simulink library "tether002_ul"  (R2020a)
settings: Solver=VariableStepAuto  StartTime=0.0  StopTime=10.0  RelTol=1e-3
values from neighbouring files (symbols this model uses):
  initNodePos = [INITIALLINE;INITIALLINE;INITIALLINE]    [tether002_ts.m]
  initNodeVel = [zeros(1,numNodes-2);zeros(1,numNodes-2);zeros(1,numNodes-2)]    [tether002_ts.m]
  numNodes = 11    [tether002_ts.m]
undefined symbols (not defined in the file or in its folder): TotoalNodes
libraries: powerlib_meascontrol x11, nodePosToLinkPos_ul x6, dspmtrx3 x4, sharedtransform x3, simulink_extras x2
(part 3 of 4)

== matlab function tether002_ul/tether001/Subsystem1/HowManyActive1 ==
  data: OriginalLengths input; ActiveNodes output; ReeledOutLength input; ActiveLengths output; TetherLength input
function [ActiveNodes, ActiveLengths] = fcn(OriginalLengths, ReeledOutLength, TetherLength)

% clc
% clear
% N = 11;
% TetherLength = 100;
% OriginalLengths = (100/(N-1))*ones(1,N-1);
% ReeledOutLength = 61;
% mid = [10,20,30,40,50,60,70,80,90;zeros(1,9);zeros(1,9)];

ActiveLengths = zeros(size(OriginalLengths));
L = zeros(size(ActiveLengths));
flag = false;
a = 1;
if ReeledOutLength == TetherLength
    L(1:end) = OriginalLengths(1:end);
else
    while flag == false
        if ReeledOutLength == sum(OriginalLengths(a:end))
            flag = true;
        elseif ReeledOutLength > sum(OriginalLengths(a:end))
            flag = true;
        else
            a=a+1;
        end
    end
L(1:end) = [zeros(1,a-2),OriginalLengths(a-1)-(sum(OriginalLengths((a-1):end))-ReeledOutLength),OriginalLengths(a:end)];
end

ActiveNodes = nnz(L)+1;
ActiveLengths = L;



% multi = 1000;
% 
% ReeledOutLength = round(ReeledOutLength*multi)/multi;
% 
% ActiveLengths = zeros(size(OriginalLengths));
% L = zeros(size(ActiveLengths));
% flag = false;
% a = 1;
% 
% if ReeledOutLength == TetherLength
%     L(1:end) = OriginalLengths(1:end);
% else
%     while flag == false
%     sumOrgLengths = round(sum(OriginalLengths(a:end))*multi)/multi;    
%         if ReeledOutLength==sumOrgLengths
%             flag = true;
%         elseif ReeledOutLength>sumOrgLengths
%             flag = true;
%         else
%             a=a+1;
%         end
%     end
% sumOrgLengthsm1 = round(sum(OriginalLengths((a-1):end))*multi)/multi;    
% L(1:end) = [zeros(1,a-2),OriginalLengths(a-1)-(sumOrgLengthsm1-ReeledOutLength),OriginalLengths(a:end)];
% end
% 
% % ReeledOutLength
% % ActiveNodesPrev
% ActiveNodes = nnz(L)+1;
% ActiveLengths = L;



% 
%[N-ActiveNodes,1,ActiveNodes-2]
%sum([N-ActiveNodes,1,N-(N-ActiveNodes+2)])

% [N-ActiveNodes+1,ActiveNodes-2,1]
% sum([N-ActiveNodes+1,ActiveNodes-2,1])

% [N-ActiveNodes,ActiveNodes-2]
% sum([N-ActiveNodes,ActiveNodes-2])


% [zeros(3,N-ActiveNodes),mid(:,(end-(ActiveNodes-3)):end)]

== matlab function tether002_ul/tether001/Subsystem1/MATLAB Function1 ==
  data: gndNodeVel input; midNodeVelInternal output; midNodeVel input; ActiveNodes input; airNodeVel input; ActiveLengths input; ReelInVel input; ReelInDirection input
function midNodeVelInternal = fcn(gndNodeVel,midNodeVel,ActiveNodes, airNodeVel, ActiveLengths, ReelInVel, ReelInDirection)

No = size(midNodeVel,2)+2;
Na = ActiveNodes;

midNodeVelInternal = [gndNodeVel(1)*ones(1,No-2);...
                      gndNodeVel(2)*ones(1,No-2);...
                      gndNodeVel(3)*ones(1,No-2)];

midNodeVelInternal(:,((No-Na)+2):end) = midNodeVel(:,((No-Na)+2):end);


nodeVelocities = [gndNodeVel,midNodeVel,airNodeVel];
linkVelocities = (nodeVelocities(:,1:end-1) + nodeVelocities(:,2:end))/2;


midNodeVelInternal(:,((No-Na)+1)) = -ReelInVel*ReelInDirection;


%midNodeVelInternal(:,((No-Na)+1)) = (linkVelocities(:,((No-Na)+1))*ActiveLengths(((No-Na)+1))+linkVelocities(:,((No-Na)+2))*ActiveLengths(((No-Na)+2)))/(ActiveLengths(((No-Na)+1))+ActiveLengths(((No-Na)+2)));




% if No == Na
%     midNodeVelInternal(:,:) = midNodeVel(:,(end-(ActiveNodes-3)):end);
% else
%     midNodeVelInternal(:,(end-(Na-3)):end) = midNodeVel(:,(end-(Na-3)):end);
% end

== matlab function tether002_ul/tether001/Subsystem1/MATLAB Function11 ==
  data: nodePos input; nodeForceVecs output; nodeVel input; ActiveLengths input; NumberNodesActive input
function nodeForceVecs = fcn(nodePos, nodeVel, ActiveLengths, NumberNodesActive)

% clc
% clear
% nodePos = [0,0,1,2,3,4,5,6,7,8,9;...
%            0,0,0,0,0,0,0,0,0,0,0;...
%            0,0,0,0,0,0,0,0,0,0,0];
% nodeVel = [1,1,1,1,0,0,0,0,0,0,0;...
%            1,1,1,1,0,0,0,0,0,0,0;...
%            1,1,1,1,0,0,0,0,0,0,0];       
% ActiveLengths = [0,0,.01,.1,.1,.1,.1,.1,.1,.1];
% NumberNodesActive = 9;
% TotalNodes = 11;

mass = .05;
zeta = .75;
diameter = .0144;
youngsMod = 5*10^10;

%Active = ActiveLengths(:,TotalNodes-NumberNodesActive+1);

TotalNodes = size(nodePos,2);

%SpringConsts = [10^7*ones(1,TotalNodes-NumberNodesActive+1),youngsMod*(pi/4)*(diameter^2)./ActiveLengths(1,(end-NumberNodesActive+3):end)];    
SpringConsts = [ones(1,TotalNodes-NumberNodesActive+1)*youngsMod*(pi/4)*(diameter^2)./ActiveLengths(1,end),youngsMod*(pi/4)*(diameter^2)./ActiveLengths(1,(end-NumberNodesActive+3):end)];    
DampCoeffs = zeta*2*sqrt(SpringConsts.*mass);

linkVecs  = diff(nodePos,1,2);

linkLength = sqrt(sum(linkVecs.^2));

linkUnitVecs = zeros(3,TotalNodes-1);
linkUnitVecs(1:3,(end-NumberNodesActive+2):end) = linkVecs(1:3,(end-NumberNodesActive+2):end)./repmat(sqrt(sum((linkVecs(1:3,(end-NumberNodesActive+2):end).^2),1)),[3 1]);

linkLengthDeriv = dot(nodeVel(:,2:end)-nodeVel(:,1:end-1),linkUnitVecs);

springForces = SpringConsts.*(linkLength-ActiveLengths);
damperForces = DampCoeffs.*linkLengthDeriv;

totalLinkForceVec = repmat(springForces+damperForces,[3 1]).*linkUnitVecs;

nodeForceVecs = [totalLinkForceVec(:,1) diff(totalLinkForceVec,1,2) -totalLinkForceVec(:,end)];

if TotalNodes~=NumberNodesActive
    nodeForceVecs(:,1) = nodeForceVecs(:,end-NumberNodesActive+1);
    nodeForceVecs(:,end-NumberNodesActive+1) = [0;0;0];
end

== matlab function tether002_ul/tether001/Subsystem1/MATLAB Function12 ==
  data: invNodeMasses output; Activelength input; ActiveNodes input
function invNodeMasses  = fcn(Activelength,ActiveNodes)
% clc
% clear
% Activelength = [0,0,.01,.1,.1,.1,.1,.1,.1,.1];
% ActiveNodes = 10;

tetherDensity = 952;
diameter = .0144;

% Mass of each link, 1xN-1
linkMasses  = tetherDensity*(Activelength*(pi/4)*diameter^2);

% 1/mass for each node, 3xN (repmat so that we can multiply with force
% vectors concatenated into matrix later
invNodeMasses = repmat(1./([linkMasses(1) linkMasses(1:end-1)+linkMasses(2:end) linkMasses(end)]/2),[3 1]);

%Make Zero Inverse mass also equal to zero
for i = 1:size(invNodeMasses,2)
    if invNodeMasses(:,i) == Inf
        invNodeMasses(:,i) = zeros(3,1);
    end
end

if invNodeMasses(:,1) == 0
    invNodeMasses(:,1) = invNodeMasses(:,end-ActiveNodes+1);
    invNodeMasses(:,end-ActiveNodes+1) = [0;0;0];
end




% REALinvNodeMasses = zeros(size(invNodeMasses));
% NonZeroRow = (find(invNodeMasses,1)+2)./3;

% if NonZeroRow>1
%     invNodeMasses(:,NonZeroRow);
%     %REALinvNodeMasses(:,1) = invNodeMasses(:,NonZeroRow);
%     %REALinvNodeMasses(:,NonZeroRow) = zeros(3,1);
% end






% tetherDensity = 952;
% diameter = .0144;
% 
% % Total Unstreched length of reeled out tether
% unstretchedLength = sum(Activelength);
% 
% % Length of each link based on active lengths 1xN-1
% linkLengths = Activelength;%linkLengths = sqrt(sum(diff(nodePos,1,2).^2));
% 
% % Total length of all links, assuming they're straight lines, scalar
% numericalTotalLength = sum(linkLengths);
% 
% % Total volume based on current tether length, scalar
% analyticalTotalVol  = unstretchedLength*(pi/4)*diameter^2;
% 
% % Total mass, based on current tether length, scalar
% analyticalTotalMass = tetherDensity*analyticalTotalVol;
% 
% % Mass of each link, 1xN-1
% linkMasses  = analyticalTotalMass*(linkLengths./numericalTotalLength);
% 
% % 1/mass for each node, 3xN (repmat so that we can multiply with force
% % vectors concatenated into matrix later
% invNodeMasses = repmat(1./([linkMasses(1) linkMasses(1:end-1)+linkMasses(2:end) linkMasses(end)]/2),[3 1]);
% 
% for i = 1:size(invNodeMasses,2)
%     if invNodeMasses(:,i) == Inf
%         invNodeMasses(:,i) = zeros(3,1);
%     end
% end
% 
% REALinvNodeMasses = zeros(size(invNodeMasses));
% NonZeroRow = (find(invNodeMasses,1)+2)./3;
% 
% if NonZeroRow>1
%     invNodeMasses(:,NonZeroRow);
%     %REALinvNodeMasses(:,1) = invNodeMasses(:,NonZeroRow);
%     %REALinvNodeMasses(:,NonZeroRow) = zeros(3,1);
% end
% 
% invNodeMasses
% end

== matlab function tether002_ul/tether001/Subsystem1/MATLAB Function13 ==
  data: nodePositions input; nodeForceVecs output; nodeVelocities input; flowVel input; NumberNodesActive input
function nodeForceVecs = fcn(nodePositions, nodeVelocities, flowVel,NumberNodesActive)
% In the notation here, N is the number of nodes, therefore you have N-1
% links between the nodes.

% N = 11;
% Length = 100;
% nodePositions = [zeros(1,N);linspace(1,Length,N);ones(1,N)];
% nodeVelocities = zeros(3,N);
% flowVel = [ones(1,N-1);.5*ones(1,N-1);.2*ones(1,N-1)];
% NumberNodesActive = 11;


flowDensity = 1025;
dragCoeff = .5;
thrDiam = .0144;

TotalNodes = size(nodePositions,2);

% Velocity and center of links 3xN-1
linkVelocities = (nodeVelocities(:,1:end-1) + nodeVelocities(:,2:end))/2;

% Apparent flow at center of links 3xN-1
linkAppFlow = flowVel - linkVelocities; %repmat(flowVel(:),[1 size(linkVelocities,2)]) - linkVelocities;
% linkAppFlow(3,:) = 0; % Origional model zeroed z component

% Link center apparent flow magnitude 3xN-1
linkAppFlowMag = sqrt(sum(linkAppFlow.^2)); % Sum over columns

% Normalize columns to get unit vector 3xN-1
dragDirUnitVec = linkAppFlow./repmat(linkAppFlowMag,[3 1]);
dragDirUnitVec(isnan(dragDirUnitVec)) = 0;

% If linkAppFlowMag is zero, dragDirUnitVec will have nans, patch to fix
% that with zeros
% dragDirUnitVec = zeros(3,numel(linkAppFlowMag==0));

% Dynamic pressures at link centers 1xN-1
dynPress = 0.5*flowDensity*linkAppFlowMag.^2;

linkVecs  = diff(nodePositions,1,2);

% Link lengths, diff over columns 1xN-1
linkLengths = sqrt(sum(diff(nodePositions,1,2).^2));

% Unit vectors in the direction of the link 3xN-1
linkUnitVecs = zeros(3,TotalNodes-1);
linkUnitVecs(1:3,(end-NumberNodesActive+2):end) = linkVecs(1:3,(end-NumberNodesActive+2):end)./repmat(sqrt(sum((linkVecs(1:3,(end-NumberNodesActive+2):end).^2),1)),[3 1]);

% Projected areas of each link
projArea = thrDiam*linkLengths.*sqrt(sum(cross(linkUnitVecs,dragDirUnitVec).^2,1));

% Drag force on links
linkForceVecs = repmat(dragCoeff*dynPress.*projArea,[3 1]).*dragDirUnitVec;

% Drag force on nodes
nodeForceVecs = [linkForceVecs(:,1) (linkForceVecs(:,1:end-1)+linkForceVecs(:,2:end)) linkForceVecs(:,end)]/2;

if NumberNodesActive<TotalNodes
    nodeForceVecs(:,1) = nodeForceVecs(:,end-NumberNodesActive+1);
    nodeForceVecs(:,end-NumberNodesActive+1) = [0;0;0];
end

== matlab function tether002_ul/tether001/Subsystem1/MATLAB Function14 ==
  data: nodePositions input; nodeForceVecs output; ActiveLengths input; NumberNodesActive input
function nodeForceVecs  = fcn(nodePositions, ActiveLengths, NumberNodesActive)

% clc
% clear
% nodePositions = [0,0,1,2,3,4,5,6,7,8,9;...
%            0,0,0,0,0,0,0,0,0,0,0;...
%            0,0,0,0,0,0,0,0,0,0,0];
%     
% ActiveLengths = [0,0,.01,.1,.1,.1,.1,.1,.1,.1];
% NumberNodesActive = 9;
% TotalNodes = 11;

tetherDensity = 952;
fluidDensity = 1025;
diameter = .0144;
gravity = 9.81;

% In this notation, N is the number of nodes

% Actual Length of each link 1xN-1
linkLengths = sqrt(sum(diff(nodePositions,1,2).^2));

% Number of links, scalar
numLinks = size(linkLengths,2);

% Volume of each link, 1xN-1
Volumes  = ActiveLengths.*(pi/4)*diameter^2;

% Mass of each link, 1xN-1
linkMasses = tetherDensity*Volumes;

% Net force on the links (buoyancy - gravity) on each link, 3xN-1
linkNetForceVecs = [repmat([0 0]',[1 numLinks]);(-gravity*linkMasses + gravity*fluidDensity*Volumes)];

% Net force on the nodes, 3xN
nodeForceVecs = [linkNetForceVecs(:,1) linkNetForceVecs(:,1:end-1)+linkNetForceVecs(:,2:end) linkNetForceVecs(:,end)]/2;

if linkMasses(1) == 0
    nodeForceVecs(:,1) = nodeForceVecs(:,end-NumberNodesActive+1);
    nodeForceVecs(:,end-NumberNodesActive+1) = [0;0;0];
end

== matlab function tether002_ul/tether001/Subsystem1/MATLAB Function15 ==
  data: gndNodePos input; midNodePosInternal output; midNodePos input; ActiveNodes input; ActiveLengths input; airNodePos input; ReelInDirection output; Na output
function [midNodePosInternal,ReelInDirection,Na] = fcn(gndNodePos, midNodePos, ActiveNodes, ActiveLengths, airNodePos)

% clc
% clear
% midNodePos = [1,2,3,4,5,6,7,8,9;...
%               1,2,3.5,4,5,6,7,8,9;...
%               1,2,3,4,5,6,7,8,9];
% ActiveLengths = [1.7,1.7,1.7,1.7,1.7,1.7,1.7,1.7,1.7];
% gndNodePos = [0;0;0];
% airNodePos = [10;10;10];
% ActiveNodes = 10;

%Radius = 15;

No = size(midNodePos,2)+2;
Na = ActiveNodes;

% if norm(midNodePos(:,(No-Na)+2))<Radius
%     Na = Na-1;
% end

% Reeled In Nodes are ground
midNodePosInternal = [gndNodePos(1)*ones(1,No-2);...
                      gndNodePos(2)*ones(1,No-2);...
                      gndNodePos(3)*ones(1,No-2)];

% Given for unalternd nodes
midNodePosInternal(:,((No-Na)+1):end) = midNodePos(:,((No-Na)+1):end);

% Find Vector between given nodes
midlinkVecs  = diff([midNodePosInternal,airNodePos],1,2);

% Find Unit Vector between given nodes
midlinkUnitVecs = midlinkVecs./repmat(sqrt(sum((midlinkVecs.^2),1)),[3 1]);

%Fixed length with slope of next link
%Option 1
ReelInDirection = midlinkUnitVecs(:,(No-Na)+1);
midNodePosInternal;


%midNodePosInternal = midNodePos;

% Fixed length with slope of to top node
% Option 2
% a = diff([gndNodePos,airNodePos],1,2);
% MULT = a./repmat(sqrt(sum((a.^2),1)),[3 1]);
% midNodePosInternal(:,((No-Na)+1)) = gndNodePos+(ActiveLengths((No-Na)+1)*MULT);
% ReelInDirection = MULT;








% if No == Na
%     %All but first the same
%     midNodePosInternal(:,2:end) = midNodePos(:,2:end);
%     %length of first unstreched slope like the second
%     midNodePosInternal(:,1) = ActiveLengths(1)*midlinkUnitVecs(:,2);
% else

== matlab function tether002_ul/tether001/Subsystem1/HowManyActive2 ==
  data: OriginalLengths input; ActiveNodes output; ReeledOutLength input; ActiveLengths output; TetherLength input; gndNodePos input; midNodePos input; airNodePos input
function [ActiveNodes, ActiveLengths] = fcn(OriginalLengths, ReeledOutLength, TetherLength,gndNodePos,midNodePos,airNodePos)

% clc
% clear
% N = 11;
% TetherLength = 100;
% OriginalLengths = (100/(N-1))*ones(1,N-1);
% ReeledOutLength = 61;
% mid = [10,20,30,40,50,60,70,80,90;zeros(1,9);zeros(1,9)];
nodePositions = [gndNodePos,midNodePos,airNodePos];
linkVecs  = diff(nodePositions,1,2);
CurrentLinkLengths = sqrt(sum(linkVecs.^2));

ActiveLengths = zeros(size(OriginalLengths));
L = zeros(size(ActiveLengths));
flag = false;
a = 1;
if ReeledOutLength == TetherLength
    a = a+1;
    %L(1:end) = OriginalLengths(1:end);
    L(1:end) = [OriginalLengths(a-1)-(sum(OriginalLengths((a-1):end))-ReeledOutLength)+(CurrentLinkLengths(a+1)-OriginalLengths(a+1))*((OriginalLengths(a-1)-(sum(OriginalLengths((a-1):end))-ReeledOutLength))/(CurrentLinkLengths(a+1))),OriginalLengths(2:end)];
else
    while flag == false
        if ReeledOutLength == sum(OriginalLengths(a:end))
            flag = true;
        elseif ReeledOutLength > sum(OriginalLengths(a:end))
            flag = true;
        else
            a=a+1;
        end
    end
    
%Org
%L(1:end) = [zeros(1,a-2),OriginalLengths(a-1)-(sum(OriginalLengths((a-1):end))-ReeledOutLength),OriginalLengths(a:end)];
    
%Weird
%L(1:end) = [zeros(1,a-2),((OriginalLengths(a-1)-(sum(OriginalLengths((a-1):end))-ReeledOutLength))-((CurrentLinkLengths(a)-(sum(CurrentLinkLengths((a):end))-ReeledOutLength)-OriginalLengths(a-1))))+(OriginalLengths(a-1)-(sum(OriginalLengths((a-1):end))-ReeledOutLength)),OriginalLengths(a:end)];

%Org+Correction
%L(1:end) = [zeros(1,a-2),OriginalLengths(a-1)-(sum(OriginalLengths((a-1):end))-ReeledOutLength)+CurrentLinkLengths(a+1)-OriginalLengths(a+1),OriginalLengths(a:end)];

%Org+Weighted Correction (Weight = (Org Length/Next Length))
L(1:end) = [zeros(1,a-2),OriginalLengths(a-1)-(sum(OriginalLengths((a-1):end))-ReeledOutLength)+(CurrentLinkLengths(a+1)-OriginalLengths(a+1))*((OriginalLengths(a-1)-(sum(OriginalLengths((a-1):end))-ReeledOutLength))/(CurrentLinkLengths(a+1))),OriginalLengths(a:end)];

% [zeros(1,a-2),CurrentLinkLengths(a:end)]
% OriginalLengths(a-1)-(sum(OriginalLengths((a-1):end))-ReeledOutLength)
% (CurrentLinkLengths(a+1)-OriginalLengths(a+1))*((OriginalLengths(a-1)-(sum(OriginalLengths((a-1):end))-ReeledOutLength))/(CurrentLinkLengths(a+1)))
end

ActiveNodes = nnz(L)+1;
ActiveLengths = L;






%CurrentLinkLengths
%OriginalLengths
% multi = 1000;
% 
% ReeledOutLength = round(ReeledOutLength*multi)/multi;
% 
% ActiveLengths = zeros(size(OriginalLengths));
% L = zeros(size(ActiveLengths));
% flag = false;
% a = 1;
% 
% if ReeledOutLength == TetherLength
%     L(1:end) = OriginalLengths(1:end);
% else
%     while flag == false
%     sumOrgLengths = round(sum(OriginalLengths(a:end))*multi)/multi;    
%         if ReeledOutLength==sumOrgLengths
%             flag = true;
%         elseif ReeledOutLength>sumOrgLengths
%             flag = true;
%         else
%             a=a+1;
%         end
%     end
% sumOrgLengthsm1 = round(sum(OriginalLengths((a-1):end))*multi)/multi;    
% L(1:end) = [zeros(1,a-2),OriginalLengths(a-1)-(sumOrgLengthsm1-ReeledOutLength),OriginalLengths(a:end)];
% end
% 
% % ReeledOutLength
% % ActiveNodesPrev
% ActiveNodes = nnz(L)+1;
% ActiveLengths = L;



% 
%[N-ActiveNodes,1,ActiveNodes-2]
%sum([N-ActiveNodes,1,N-(N-ActiveNodes+2)])

% [N-ActiveNodes+1,ActiveNodes-2,1]
% sum([N-ActiveNodes+1,ActiveNodes-2,1])

% [N-ActiveNodes,ActiveNodes-2]
% sum([N-ActiveNodes,ActiveNodes-2])


% [zeros(3,N-ActiveNodes),mid(:,(end-(ActiveNodes-3)):end)]

== matlab function tether002_ul/tether001/Subsystem1/MATLAB Function16 ==
  data: gndNodeVel input; midNodeVelInternal output; midNodeVel input; ActiveNodes input; airNodeVel input; ActiveLengths input; ReelInVel input; ReelInDirection input
function midNodeVelInternal = fcn(gndNodeVel,midNodeVel,ActiveNodes, airNodeVel, ActiveLengths, ReelInVel, ReelInDirection)

No = size(midNodeVel,2)+2;
Na = ActiveNodes;

midNodeVelInternal = [gndNodeVel(1)*ones(1,No-2);...
                      gndNodeVel(2)*ones(1,No-2);...
                      gndNodeVel(3)*ones(1,No-2)];

midNodeVelInternal(:,((No-Na)+2):end) = midNodeVel(:,((No-Na)+2):end);


nodeVelocities = [gndNodeVel,midNodeVel,airNodeVel];
linkVelocities = (nodeVelocities(:,1:end-1) + nodeVelocities(:,2:end))/2;


midNodeVelInternal(:,((No-Na)+1)) = -ReelInVel*ReelInDirection;


%midNodeVelInternal(:,((No-Na)+1)) = (linkVelocities(:,((No-Na)+1))*ActiveLengths(((No-Na)+1))+linkVelocities(:,((No-Na)+2))*ActiveLengths(((No-Na)+2)))/(ActiveLengths(((No-Na)+1))+ActiveLengths(((No-Na)+2)));




% if No == Na
%     midNodeVelInternal(:,:) = midNodeVel(:,(end-(ActiveNodes-3)):end);
% else
%     midNodeVelInternal(:,(end-(Na-3)):end) = midNodeVel(:,(end-(Na-3)):end);
% end

== matlab function tether002_ul/tether001/Subsystem1/MATLAB Function17 ==
  data: nodePos input; nodeForceVecs output; nodeVel input; ActiveLengths input; NumberNodesActive input; linkLength output
function [nodeForceVecs,linkLength] = fcn(nodePos, nodeVel, ActiveLengths, NumberNodesActive)

% clc
% clear
% nodePos = [0,0,1,2,3,4,5,6,7,8,9;...
%            0,0,0,0,0,0,0,0,0,0,0;...
%            0,0,0,0,0,0,0,0,0,0,0];
% nodeVel = [1,1,1,1,0,0,0,0,0,0,0;...
%            1,1,1,1,0,0,0,0,0,0,0;...
%            1,1,1,1,0,0,0,0,0,0,0];       
% ActiveLengths = [0,0,.01,.1,.1,.1,.1,.1,.1,.1];
% NumberNodesActive = 9;
% TotalNodes = 11;

mass = .05;
zeta = .75;
diameter = .0144;
youngsMod = 5*10^10;

%Active = ActiveLengths(:,TotalNodes-NumberNodesActive+1);

TotalNodes = size(nodePos,2);

SpringConsts = [zeros(1,TotalNodes-NumberNodesActive+1),youngsMod*(pi/4)*(diameter^2)./ActiveLengths(1,(end-NumberNodesActive+3):end)];
DampCoeffs = zeta*2*sqrt(SpringConsts.*mass);

linkVecs  = diff(nodePos,1,2);

linkLength = sqrt(sum(linkVecs.^2));

linkUnitVecs = zeros(3,TotalNodes-1);
linkUnitVecs(1:3,(end-NumberNodesActive+2):end) = linkVecs(1:3,(end-NumberNodesActive+2):end)./repmat(sqrt(sum((linkVecs(1:3,(end-NumberNodesActive+2):end).^2),1)),[3 1]);

linkLengthDeriv = dot(nodeVel(:,2:end)-nodeVel(:,1:end-1),linkUnitVecs);

springForces = SpringConsts.*(linkLength-ActiveLengths);
damperForces = DampCoeffs.*linkLengthDeriv;

totalLinkForceVec = repmat(springForces+damperForces,[3 1]).*linkUnitVecs;

nodeForceVecs = [totalLinkForceVec(:,1) diff(totalLinkForceVec,1,2) -totalLinkForceVec(:,end)];

if SpringConsts(1) == 0
    nodeForceVecs(:,1) = nodeForceVecs(:,end-NumberNodesActive+2);
    nodeForceVecs(:,end-NumberNodesActive+2) = [0;0;0];
end
2;
nodeForceVecs;

== matlab function tether002_ul/tether001/Subsystem1/MATLAB Function18 ==
  data: invNodeMasses output; Activelength input; ActiveNodes input
function invNodeMasses  = fcn(Activelength,ActiveNodes)
% clc
% clear
% Activelength = [0,0,.01,.1,.1,.1,.1,.1,.1,.1];
% ActiveNodes = 10;

tetherDensity = 952;
diameter = .0144;

Na = ActiveNodes;
No = length(Activelength)+1;

% Mass of each link, 1xN-1
linkMasses  = tetherDensity*(Activelength*(pi/4)*diameter^2);

% 1/mass for each node, 3xN (repmat so that we can multiply with force
% vectors concatenated into matrix later
invNodeMasses = zeros(3,No);
invNodeMasses(:,(No-Na+1):end) = repmat(1./([linkMasses((No-Na+1)) linkMasses((No-Na+1):end-1)+linkMasses((No-Na+2):end) linkMasses(end)]/2),[3 1]);

%Make Zero Inverse mass also equal to zero
for i = 1:size(invNodeMasses,2)
    if invNodeMasses(:,i) == Inf
        invNodeMasses(:,i) = zeros(3,1);
    end
end

% if invNodeMasses(:,1) == 0
%     invNodeMasses(:,1) = invNodeMasses(:,end-ActiveNodes+1);
%     invNodeMasses(:,end-ActiveNodes+1) = [0;0;0];
% end



% REALinvNodeMasses = zeros(size(invNodeMasses));
% NonZeroRow = (find(invNodeMasses,1)+2)./3;

% if NonZeroRow>1
%     invNodeMasses(:,NonZeroRow);
%     %REALinvNodeMasses(:,1) = invNodeMasses(:,NonZeroRow);
%     %REALinvNodeMasses(:,NonZeroRow) = zeros(3,1);
% end






% tetherDensity = 952;
% diameter = .0144;
% 
% % Total Unstreched length of reeled out tether
% unstretchedLength = sum(Activelength);
% 
% % Length of each link based on active lengths 1xN-1
% linkLengths = Activelength;%linkLengths = sqrt(sum(diff(nodePos,1,2).^2));
% 
% % Total length of all links, assuming they're straight lines, scalar
% numericalTotalLength = sum(linkLengths);
% 
% % Total volume based on current tether length, scalar
% analyticalTotalVol  = unstretchedLength*(pi/4)*diameter^2;
% 
% % Total mass, based on current tether length, scalar
% analyticalTotalMass = tetherDensity*analyticalTotalVol;
% 
% % Mass of each link, 1xN-1
% linkMasses  = analyticalTotalMass*(linkLengths./numericalTotalLength);
% 
% % 1/mass for each node, 3xN (repmat so that we can multiply with force
% % vectors concatenated into matrix later
% invNodeMasses = repmat(1./([linkMasses(1) linkMasses(1:end-1)+linkMasses(2:end) linkMasses(end)]/2),[3 1]);
% 
% for i = 1:size(invNodeMasses,2)
%     if invNodeMasses(:,i) == Inf
%         invNodeMasses(:,i) = zeros(3,1);
%     end
% end
% 
% REALinvNodeMasses = zeros(size(invNodeMasses));
% NonZeroRow = (find(invNodeMasses,1)+2)./3;
% 
% if NonZeroRow>1
%     invNodeMasses(:,NonZeroRow);
%     %REALinvNodeMasses(:,1) = invNodeMasses(:,NonZeroRow);
%     %REALinvNodeMasses(:,NonZeroRow) = zeros(3,1);
% end
% 
% invNodeMasses
% end

== matlab function tether002_ul/tether001/Subsystem1/MATLAB Function19 ==
  data: nodePositions input; nodeForceVecs output; nodeVelocities input; flowVel input; NumberNodesActive input
function nodeForceVecs = fcn(nodePositions, nodeVelocities, flowVel,NumberNodesActive)
% In the notation here, N is the number of nodes, therefore you have N-1
% links between the nodes.

% N = 11;
% Length = 100;
% nodePositions = [zeros(1,N);linspace(1,Length,N);ones(1,N)];
% nodeVelocities = zeros(3,N);
% flowVel = [ones(1,N-1);.5*ones(1,N-1);.2*ones(1,N-1)];
% NumberNodesActive = 11;


flowDensity = 1025;
dragCoeff = .5;
thrDiam = .0144;

TotalNodes = size(nodePositions,2);

% Velocity and center of links 3xN-1
linkVelocities = (nodeVelocities(:,1:end-1) + nodeVelocities(:,2:end))/2;

% Apparent flow at center of links 3xN-1
linkAppFlow = flowVel - linkVelocities; %repmat(flowVel(:),[1 size(linkVelocities,2)]) - linkVelocities;
% linkAppFlow(3,:) = 0; % Origional model zeroed z component

% Link center apparent flow magnitude 3xN-1
linkAppFlowMag = sqrt(sum(linkAppFlow.^2)); % Sum over columns

% Normalize columns to get unit vector 3xN-1
dragDirUnitVec = linkAppFlow./repmat(linkAppFlowMag,[3 1]);
dragDirUnitVec(isnan(dragDirUnitVec)) = 0;

% If linkAppFlowMag is zero, dragDirUnitVec will have nans, patch to fix
% that with zeros
% dragDirUnitVec = zeros(3,numel(linkAppFlowMag==0));

% Dynamic pressures at link centers 1xN-1
dynPress = 0.5*flowDensity*linkAppFlowMag.^2;

linkVecs  = diff(nodePositions,1,2);

% Link lengths, diff over columns 1xN-1
linkLengths = sqrt(sum(diff(nodePositions,1,2).^2));

% Unit vectors in the direction of the link 3xN-1
linkUnitVecs = zeros(3,TotalNodes-1);
linkUnitVecs(1:3,(end-NumberNodesActive+2):end) = linkVecs(1:3,(end-NumberNodesActive+2):end)./repmat(sqrt(sum((linkVecs(1:3,(end-NumberNodesActive+2):end).^2),1)),[3 1]);

% Projected areas of each link
projArea = thrDiam*linkLengths.*sqrt(sum(cross(linkUnitVecs,dragDirUnitVec).^2,1));

% Drag force on links
linkForceVecs = repmat(dragCoeff*dynPress.*projArea,[3 1]).*dragDirUnitVec;

% Drag force on nodes
nodeForceVecs = zeros(3,TotalNodes);
nodeForceVecs(:,(TotalNodes-NumberNodesActive+1):end) = [linkForceVecs(:,(TotalNodes-NumberNodesActive+1)), (linkForceVecs(:,((TotalNodes-NumberNodesActive+1)):end-1)+linkForceVecs(:,((TotalNodes-NumberNodesActive+2)):end)) linkForceVecs(:,end)]/2;


if NumberNodesActive<TotalNodes
    nodeForceVecs(:,1) = nodeForceVecs(:,end-NumberNodesActive+1);
    nodeForceVecs(:,end-NumberNodesActive+1) = [0;0;0];
end

== matlab function tether002_ul/tether001/Subsystem1/MATLAB Function20 ==
  data: nodePositions input; nodeForceVecs output; ActiveLengths input; NumberNodesActive input
function nodeForceVecs  = fcn(nodePositions, ActiveLengths, NumberNodesActive)

% clc
% clear
% nodePositions = [0,0,1,2,3,4,5,6,7,8,9;...
%            0,0,0,0,0,0,0,0,0,0,0;...
%            0,0,0,0,0,0,0,0,0,0,0];
%     
% ActiveLengths = [0,0,.01,.1,.1,.1,.1,.1,.1,.1];
% NumberNodesActive = 9;
% TotalNodes = 11;

tetherDensity = 952;
fluidDensity = 1025;
diameter = .0144;
gravity = 9.81;

% In this notation, N is the number of nodes

% Actual Length of each link 1xN-1
linkLengths = sqrt(sum(diff(nodePositions,1,2).^2));

% Number of links, scalar
numLinks = size(linkLengths,2);

% Volume of each link, 1xN-1
Volumes  = ActiveLengths.*(pi/4)*diameter^2;

% Mass of each link, 1xN-1
linkMasses = tetherDensity*Volumes;

% Net force on the links (buoyancy - gravity) on each link, 3xN-1
linkNetForceVecs = [repmat([0 0]',[1 numLinks]);(-gravity*linkMasses + gravity*fluidDensity*Volumes)];

% Net force on the nodes, 3xN
nodeForceVecs = [linkNetForceVecs(:,1) linkNetForceVecs(:,1:end-1)+linkNetForceVecs(:,2:end) linkNetForceVecs(:,end)]/2;

if linkMasses(1) == 0
    nodeForceVecs(:,1) = nodeForceVecs(:,end-NumberNodesActive+2);
    nodeForceVecs(:,end-NumberNodesActive+2) = [0;0;0];
end
3;
nodeForceVecs;

== matlab function tether002_ul/tether001/Subsystem1/MATLAB Function21 ==
  data: gndNodePos input; midNodePosInternal output; midNodePos input; ActiveNodes input; ActiveLengths input; airNodePos input; ReelInDirection output; Na output
function [midNodePosInternal,ReelInDirection,Na] = fcn(gndNodePos, midNodePos, ActiveNodes, ActiveLengths, airNodePos)

% clc
% clear
% midNodePos = [1,2,3,4,5,6,7,8,9;...
%               1,2,3.5,4,5,6,7,8,9;...
%               1,2,3,4,5,6,7,8,9];
% ActiveLengths = [1.7,1.7,1.7,1.7,1.7,1.7,1.7,1.7,1.7];
% gndNodePos = [0;0;0];
% airNodePos = [10;10;10];
% ActiveNodes = 10;

%Radius = 15;

No = size(midNodePos,2)+2;
Na = ActiveNodes;

% if norm(midNodePos(:,(No-Na)+2))<Radius
%     Na = Na-1;
% end

% Reeled In Nodes are ground
midNodePosInternal = [gndNodePos(1)*ones(1,No-2);...
                      gndNodePos(2)*ones(1,No-2);...
                      gndNodePos(3)*ones(1,No-2)];

% Given for unalternd nodes
midNodePosInternal(:,((No-Na)+2):end) = midNodePos(:,((No-Na)+2):end);

% Find Vector between given nodes
midlinkVecs  = diff([midNodePosInternal,airNodePos],1,2);
TotalVec = diff([gndNodePos,airNodePos],1,2);

% Find Unit Vector between given nodes
midlinkUnitVecs = midlinkVecs./repmat(sqrt(sum((midlinkVecs.^2),1)),[3 1]);
TotalUnitVec = TotalVec./repmat(sqrt(sum((TotalVec.^2),1)),[3 1]);



% %Fixed length with slope of next link
% %Option 1
midNodePosInternal(:,((No-Na)+1)) = gndNodePos+(ActiveLengths((No-Na)+1)*midlinkUnitVecs(:,(No-Na)+1));
ReelInDirection = midlinkUnitVecs(:,(No-Na)+1);

% Fixed length with slope of to top node
% Option 2
% a = diff([gndNodePos,airNodePos],1,2);
% MULT = a./repmat(sqrt(sum((a.^2),1)),[3 1]);
% midNodePosInternal(:,((No-Na)+1)) = gndNodePos+(ActiveLengths((No-Na)+1)*MULT);
% ReelInDirection = MULT;


%Matching 1-2 and 2-3 Angle
% %Option 3
% r_A = TotalUnitVec(:,1);
% r_C = midlinkUnitVecs(:,(No-Na)+1);
% r_D = midlinkUnitVecs(:,(No-Na)+2);
% 
% if ne(r_D,r_C)
%     v = cross(r_D,r_C); 
%     ssc = [0 -v(3) v(2); v(3) 0 -v(1); -v(2) v(1) 0]; 
%     C_c_D = eye(3) + ssc + ssc^2*(1-dot(r_D,r_C))/(norm(v))^2;
% else
%     C_c_D = eye(3);
% end
% D_c_C = C_c_D';
% 
% if ne(r_A,r_D)
%     v = cross(r_A,r_D); 
%     ssc = [0 -v(3) v(2); v(3) 0 -v(1); -v(2) v(1) 0]; 
%     D_c_A = eye(3) + ssc + ssc^2*(1-dot(r_A,r_D))/(norm(v))^2;    
% else
%     D_c_A = eye(3);
% end
% A_c_D = D_c_A';
% 
% C_c_A = C_c_D*D_c_A;
% 
% B_c_C = C_c_D;
% 
% B_c_A = C_c_A;
% 
% midNodePosInternal(:,((No-Na)+1)) = gndNodePos + ActiveLengths((No-Na)+1)*(B_c_A*r_A);
% ReelInDirection = (B_c_A*midlinkUnitVecs(:,(No-Na)+1));







































%BAD%Option 
% H1 = diff([gndNodePos,airNodePos],1,2);
% H = H1./repmat(sqrt(sum((H1.^2),1)),[3 1]);
% 
% A = midlinkUnitVecs(:,(No-Na)+1);
% B = midlinkUnitVecs(:,(No-Na)+2);
% if A~=B
%     %%%%%%
%     G = [ dot(A,B) -norm(cross(A,B)) 0;...
%          norm(cross(A,B)) dot(A,B)  0;...
%          0              0           1];
%     Fi = [ A (B-dot(A,B)*A)/norm(B-dot(A,B)*A) cross(B,A) ];
%     B2_C_B3 = Fi*G*inv(Fi);
%     %%%%%%
%     Q = [ dot(H,A) -norm(cross(H,A)) 0;...
%      norm(cross(H,A)) dot(H,A)  0;...
%      0              0           1];
%     Qi = [ H (A-dot(H,A)*H)/norm(A-dot(H,A)*H) cross(A,H) ];
%     B1_C_B3 = Qi*Q*inv(Qi);
%     B1_C_B3 = B1_C_B3*B2_C_B3';
%     
%     midNodePosInternal(:,((No-Na)+1)) = gndNodePos + ActiveLengths((No-Na)+1)*(B1_C_B3*midlinkUnitVecs(:,(No-Na)+1));
%     ReelInDirection = (B1_C_B3*midlinkUnitVecs(:,(No-Na)+1));
% else
%     midNodePosInternal(:,((No-Na)+1)) = gndNodePos + ActiveLengths((No-Na)+1)*(midlinkUnitVecs(:,(No-Na)+1));
%     ReelInDirection = midlinkUnitVecs(:,(No-Na)+1);
% end











% if No == Na
%     %All but first the same
%     midNodePosInternal(:,2:end) = midNodePos(:,2:end);
%     %length of first unstreched slope like the second
%     midNodePosInternal(:,1) = ActiveLengths(1)*midlinkUnitVecs(:,2);
% else

== matlab function tether002_ul/tether001/Subsystem1/MATLAB Function22 ==
  data: nodePositions input; CurrentLinkLengthss output
function CurrentLinkLengthss = fcn(nodePositions)

linkVecss  = diff(nodePositions,1,2);
CurrentLinkLengthss = sqrt(sum(linkVecss.^2));

== matlab function tether002_ul/tether001/HowManyActive3 ==
  data: OriginalLengths input; ActiveNodes output; ReeledOutLength input; ActiveLengths output; TetherLength input; OriginalNodes output; Lcorrected input; ActiveLengthsUncorrected output; Scope output
function [ActiveNodes, ActiveLengths, OriginalNodes,ActiveLengthsUncorrected, Scope]= fcn(OriginalLengths, ReeledOutLength, TetherLength, Lcorrected)%, r_BA, r_AO)

%Prealocate and set initial counter and boolean
ActiveLengths = zeros(size(OriginalLengths));
L = zeros(size(ActiveLengths));
Lunc = zeros(size(ActiveLengths));
flag = false;
a = 1;

%Tether cant be reeled out past max length
if ReeledOutLength>TetherLength
    ReeledOutLength = TetherLength;
end

%Finds out link lenghts based on tether length
if ReeledOutLength == TetherLength %Fully reeled out
    a = a+1;
    L(1:end) = OriginalLengths(1:end);
    Lunc(1:end) = OriginalLengths(1:end);
else
    while flag == false
        if ReeledOutLength == sum(OriginalLengths(a:end))
            flag = true;
        elseif ReeledOutLength > sum(OriginalLengths(a:end))
            flag = true;
        else
            a=a+1;
        end
    end
    
    %If not on last link
    if ReeledOutLength>OriginalLengths(1)
        if Lcorrected<OriginalLengths(a)
            Lcorrected = OriginalLengths(a);
        end
        if Lcorrected==0 %No Correction
            L(1:end) = [zeros(1,a-2),OriginalLengths(a-1)-(sum(OriginalLengths((a-1):end))-ReeledOutLength),OriginalLengths(a:end)];
            Lunc(1:end) = [zeros(1,a-2),OriginalLengths(a-1)-(sum(OriginalLengths((a-1):end))-ReeledOutLength),OriginalLengths(a:end)];        
        elseif a <= length(OriginalLengths)-1
            L(1:end) = [zeros(1,a-2),OriginalLengths(a-1)-(sum(OriginalLengths((a-1):end))-ReeledOutLength)+(Lcorrected-OriginalLengths(a+1))*((OriginalLengths(a-1)-(sum(OriginalLengths((a-1):end))-ReeledOutLength))/(Lcorrected)),OriginalLengths(a:end)];
            Lunc(1:end) = [zeros(1,a-2),OriginalLengths(a-1)-(sum(OriginalLengths((a-1):end))-ReeledOutLength),OriginalLengths(a:end)];        
        else
        	L(1:end) = [zeros(1,a-2),OriginalLengths(a-1)-(sum(OriginalLengths((a-1):end))-ReeledOutLength)+(Lcorrected-OriginalLengths(end))*((OriginalLengths(a-1)-(sum(OriginalLengths((a-1):end))-ReeledOutLength))/(Lcorrected)),OriginalLengths(a:end)];    
        	Lunc(1:end) = [zeros(1,a-2),OriginalLengths(a-1)-(sum(OriginalLengths((a-1):end))-ReeledOutLength),OriginalLengths(a:end)];    
        end
    %on last link
    else
        if Lcorrected<OriginalLengths(end)
            Lcorrected = OriginalLengths(end);
        end
        L(end) = ReeledOutLength+(Lcorrected-OriginalLengths(end))*((OriginalLengths(a-1)-(sum(OriginalLengths((a-1):end))-ReeledOutLength))/(Lcorrected));
        Lunc(end) = ReeledOutLength;    
    end

end

% Active Nodes include ground, air, and nodes not reeled in
% for example if 74m of 11  (including ground and air) node 
% 100m tether are reeled out there will be 9 "Active Nodes"
ActiveNodes = nnz(L)+1;

%Active lengths is a 1xN-1 length row vector where 
ActiveLengths = L;
OriginalNodes = length(OriginalLengths)+1;


ActiveLengthsUncorrected = Lunc;



Scope = Lcorrected;


    %L(1:end) = [OriginalLengths(a-1)-(sum(OriginalLengths((a-1):end))-ReeledOutLength)+(CurrentLinkLengths(a+1)-OriginalLengths(a+1))*((OriginalLengths(a-1)-(sum(OriginalLengths((a-1):end))-ReeledOutLength))/(CurrentLinkLengths(a+1))),OriginalLengths(2:end)];
    %L(1:end) = [OriginalLengths(a-1)-(sum(OriginalLengths((a-1):end))-ReeledOutLength)+(CurrentLinkLengths-OriginalLengths(a+1))*((OriginalLengths(a-1)-(sum(OriginalLengths((a-1):end))-ReeledOutLength))/(CurrentLinkLengths)),OriginalLengths(2:end)];



%Remove!! Just for test%%%%%%%%%%%5
% if ReeledOutLength<=.1
%     ReeledOutLength = TetherLength;
% end

        % %Org
        % L(1:end) = [zeros(1,a-2),OriginalLengths(a-1)-(sum(OriginalLengths((a-1):end))-ReeledOutLength),OriginalLengths(a:end)];

        % %Org Corrected

        


            %         else
%             L(1:end) = [zeros(1,a-2),OriginalLengths(a-1)-(sum(OriginalLengths((a-1):end))-ReeledOutLength)+(Lcorrected-              0)*((OriginalLengths(a-1)-(sum(OriginalLengths((a-1):end))-ReeledOutLength))/(Lcorrected)),OriginalLengths(a:end)]    
%         end

        %Radius + -
        % L(1:end) = [zeros(1,a-2),OriginalLengths(a-1)-(sum(OriginalLengths((a-1):end))-ReeledOutLength)+Radius,OriginalLengths(a)-Radius,OriginalLengths(a+1:end)];   

        %Radius +
        %L(1:end) = [zeros(1,a-2),OriginalLengths(a-1)-(sum(OriginalLengths((a-1):end))-ReeledOutLength)+Radius,OriginalLengths(a:end)];   
        
        %Weird
        %L(1:end) = [zeros(1,a-2),((OriginalLengths(a-1)-(sum(OriginalLengths((a-1):end))-ReeledOutLength))-((CurrentLinkLengths(a)-(sum(CurrentLinkLengths((a):end))-ReeledOutLength)-OriginalLengths(a-1))))+(OriginalLengths(a-1)-(sum(OriginalLengths((a-1):end))-ReeledOutLength)),OriginalLengths(a:end)];

        %Org+Correction
        %L(1:end) = [zeros(1,a-2),OriginalLengths(a-1)-(sum(OriginalLengths((a-1):end))-ReeledOutLength)+CurrentLinkLengths(a+1)-OriginalLengths(a+1),OriginalLengths(a:end)];

        %Org+Weighted Correction (Weight = (Org Length/Next Length))
        %L(1:end) = [zeros(1,a-2),OriginalLengths(a-1)-(sum(OriginalLengths((a-1):end))-ReeledOutLength)+(CurrentLinkLengths(a+1)-OriginalLengths(a+1))*((OriginalLengths(a-1)-(sum(OriginalLengths((a-1):end))-ReeledOutLength))/(CurrentLinkLengths(a+1))),OriginalLengths(a:end)];
        %L(1:end) = [zeros(1,a-2),OriginalLengths(a-1)-(sum(OriginalLengths((a-1):end))-ReeledOutLength)+(CurrentLinkLengths-OriginalLengths(a+1))*((OriginalLengths(a-1)-(sum(OriginalLengths((a-1):end))-ReeledOutLength))/(CurrentLinkLengths)),OriginalLengths(a:end)];


        % [zeros(1,a-2),CurrentLinkLengths(a:end)]
        % OriginalLengths(a-1)-(sum(OriginalLengths((a-1):end))-ReeledOutLength)
        % (CurrentLinkLengths(a+1)-OriginalLengths(a+1))*((OriginalLengths(a-1)-(sum(OriginalLengths((a-1):end))-ReeledOutLength))/(CurrentLinkLengths(a+1)))
    
% clc
% clear
% N = 11;
% TetherLength = 100;
% OriginalLengths = (100/(N-1))*ones(1,N-1);
% ReeledOutLength = 61;
% mid = [10,20,30,40,50,60,70,80,90;zeros(1,9);zeros(1,9)];
% 
%fcn(OriginalLengths, ReeledOutLength, TetherLength,gndNodePos,midNodePos,airNodePos)
% nodePositions = [gndNodePos,midNodePos,airNodePos];
% linkVecs  = diff(nodePositions,1,2);
% CurrentLinkLengths = sqrt(sum(linkVecs.^2));

%CurrentLinkLengths = norm(r_BA);
%Radius = .1;



%CurrentLinkLengths
%OriginalLengths
% multi = 1000;
% 
% ReeledOutLength = round(ReeledOutLength*multi)/multi;
% 
% ActiveLengths = zeros(size(OriginalLengths));
% L = zeros(size(ActiveLengths));
% flag = false;
% a = 1;
% 
% if ReeledOutLength == TetherLength
%     L(1:end) = OriginalLengths(1:end);
% else
%     while flag == false
%     sumOrgLengths = round(sum(OriginalLengths(a:end))*multi)/multi;    
%         if ReeledOutLength==sumOrgLengths
%             flag = true;
%         elseif ReeledOutLength>sumOrgLengths
%             flag = true;
%         else
%             a=a+1;
%         end
%     end
% sumOrgLengthsm1 = round(sum(OriginalLengths((a-1):end))*multi)/multi;    
% L(1:end) = [zeros(1,a-2),OriginalLengths(a-1)-(sumOrgLengthsm1-ReeledOutLength),OriginalLengths(a:end)];
% end
% 
% % ReeledOutLength
% % ActiveNodesPrev
% ActiveNodes = nnz(L)+1;
% ActiveLengths = L;



% 
%[N-ActiveNodes,1,ActiveNodes-2]
%sum([N-ActiveNodes,1,N-(N-ActiveNodes+2)])

% [N-ActiveNodes+1,ActiveNodes-2,1]
% sum([N-ActiveNodes+1,ActiveNodes-2,1])

% [N-ActiveNodes,ActiveNodes-2]
% sum([N-ActiveNodes,ActiveNodes-2])


% [zeros(3,N-ActiveNodes),mid(:,(end-(ActiveNodes-3)):end)]

== matlab function tether002_ul/tether001/Subsystem1/Tension/MATLAB Function ==
  data: nodePositions input; nodeForceVecs output; nodeVelocities input; unstretchedLength input
function nodeForceVecs = nodeSpringDamperForce(nodePositions,nodeVelocities,unstretchedLength)

mass = .05;
zeta = .75;
diameter = .0144;
youngsMod = 50*10^9;

% Number of nodes
N = size(nodePositions,2);

% total spring stiffness
totalSpringConst = youngsMod*(pi/4)*(diameter^2)/unstretchedLength;

% total damping coefficient
totalDampCoeff = zeta*2*sqrt(totalSpringConst*mass);

% Spring constant and damping coefficient for each link
linkSpringConst  = totalSpringConst*(N-1);
linkDampingCoeff = totalDampCoeff*(N-1);
meanLinkLength   = unstretchedLength/(N-1);

% Vector from one node to another
linkVecs  = diff(nodePositions,1,2);

% Length of each link
linkLength = sqrt(sum(linkVecs.^2));

% Link direction unit vectors
linkUnitVecs = linkVecs./repmat(sqrt(sum(linkVecs.^2,1)),[3 1]);

% Rate of change of vector from one node to another
linkLengthDeriv = dot(nodeVelocities(:,2:end)-nodeVelocities(:,1:end-1),linkUnitVecs);


% Magnitude of spring force on each link
springForces = zeros(size(linkLength));
springForces(linkLength>meanLinkLength) = linkSpringConst*(linkLength(linkLength>meanLinkLength)-meanLinkLength);

% Magnitude of damping force on each link
damperForces  = zeros(size(linkLengthDeriv));
damperForces(linkLength>meanLinkLength) = linkDampingCoeff*linkLengthDeriv(linkLength>meanLinkLength);

% Total force in each link
totalLinkForceVec = repmat(springForces+damperForces,[3 1]).*linkUnitVecs;

% Force on each node
nodeForceVecs = [totalLinkForceVec(:,1) diff(totalLinkForceVec,1,2) -totalLinkForceVec(:,end)];

end

== matlab function tether002_ul/tether001/MATLAB Function39 ==
  data: ReeledOutLength input; nodePos input; nodeForceVecs output size=[3,numNodes]; nodeVel input; ActiveLengths input; NumberNodesActive input
function nodeForceVecs  = fcn(ReeledOutLength, nodePos, nodeVel, ActiveLengths, NumberNodesActive)

% clc
% clear
% nodePos = [0,0,1,2,3,4,5,6,7,8,9;...
%            0,0,0,0,0,0,0,0,0,0,0;...
%            0,0,0,0,0,0,0,0,0,0,0];
% nodeVel = [1,1,1,1,0,0,0,0,0,0,0;...
%            1,1,1,1,0,0,0,0,0,0,0;...
%            1,1,1,1,0,0,0,0,0,0,0];       
% ActiveLengths = [0,0,.01,.1,.1,.1,.1,.1,.1,.1];
% NumberNodesActive = 9;
% TotalNodes = 11;

mass = .05;
zeta = .75;
diameter = .0144;
youngsMod = 5*10^10;

%Active = ActiveLengths(:,TotalNodes-NumberNodesActive+1);
unstretchedLength = ReeledOutLength;
totalSpringConst = youngsMod*(pi/4)*(diameter^2)/unstretchedLength;

%Test
if totalSpringConst == Inf || totalSpringConst>10^9
    totalSpringConst = 10^9;
end

TotalNodes = size(nodePos,2);
No = TotalNodes;
Na = NumberNodesActive;
LengthActive = ActiveLengths(1,(No-Na+1));

MatchedSpringConst = totalSpringConst*(Na-2);

SpringConsts = zeros(1,TotalNodes-1);

if Na>2
    %Non-Preserve
    SpringConsts(:,(No-Na+2):end) = youngsMod*(pi/4)*(diameter^2)./ActiveLengths(1,(end-NumberNodesActive+3):end);
    %SpringConsts = [zeros(1,TotalNodes-NumberNodesActive+1),youngsMod*(pi/4)*(diameter^2)./ActiveLengths(1,(end-NumberNodesActive+3):end)];
    
    %Preserve
    %SpringConsts(:,(No-Na+2):end) = MatchedSpringConst*ones(size(ActiveLengths(1,(No-Na+2):end)));
    %SpringConsts = [zeros(1,TotalNodes-NumberNodesActive+1),MatchedSpringConst*ones(size(ActiveLengths(1,(No-Na+2):end)))];
else
    SpringConsts(end) = totalSpringConst;
end

DampCoeffs = zeta*2*sqrt(SpringConsts.*mass);


a = zeros(1,length(SpringConsts));
for i = 1:length(SpringConsts)
    if SpringConsts(i)==0
        a(i) = 0;
    else
        a(i) = 1/SpringConsts(i);
    end
end
1/sum(a);


linkVecs  = diff(nodePos,1,2);

linkLength = sqrt(sum(linkVecs.^2));

linkUnitVecs = zeros(3,TotalNodes-1);
linkUnitVecs(1:3,(end-NumberNodesActive+2):end) = linkVecs(1:3,(end-NumberNodesActive+2):end)./repmat(sqrt(sum((linkVecs(1:3,(end-NumberNodesActive+2):end).^2),1)),[3 1]);

linkLengthDeriv = dot(nodeVel(:,2:end)-nodeVel(:,1:end-1),linkUnitVecs);

Active = ActiveLengths;
Comb = linkLength-ActiveLengths;

springForces = SpringConsts.*(linkLength-ActiveLengths);
damperForces = DampCoeffs.*linkLengthDeriv;

totalLinkForceVec = repmat(springForces+damperForces,[3 1]).*linkUnitVecs;

nodeForceVecs = [totalLinkForceVec(:,1) diff(totalLinkForceVec,1,2) -totalLinkForceVec(:,end)];

if SpringConsts(1) == 0
    nodeForceVecs(:,1) = nodeForceVecs(:,No-Na+1);
    nodeForceVecs(:,No-Na+1) = [0;0;0];
% elseif SpringConsts(end) == totalSpringConst
%     nodeForceVecs(:,No-Na+1) = nodeForceVecs(:,1);
%     nodeForceVecs(:,1) = [0;0;0];
end


% 1
%SPRING

== matlab function tether002_ul/tether001/MATLAB Function40 ==
  data: invNodeMasses output size=[3,numNodes]; Activelength input; ActiveNodes input
function invNodeMasses  = fcn(Activelength,ActiveNodes)
% clc
% clear
% Activelength = [0,0,.01,.1,.1,.1,.1,.1,.1,.1];
% ActiveNodes = 10;

tetherDensity = 952;
diameter = .0144;

Na = ActiveNodes;
No = length(Activelength)+1;

% Mass of each link, 1xN-1
linkMasses  = tetherDensity*(Activelength*(pi/4)*diameter^2);

% 1/mass for each node, 3xN (repmat so that we can multiply with force
% vectors concatenated into matrix later
invNodeMasses = zeros(3,No);
invNodeMasses(:,(No-Na+1):end) = repmat(1./([linkMasses((No-Na+1)) linkMasses((No-Na+1):end-1)+linkMasses((No-Na+2):end) linkMasses(end)]/2),[3 1]);

%Make Zero Inverse mass also equal to zero
for i = 1:size(invNodeMasses,2)
    if invNodeMasses(:,i) == Inf
        invNodeMasses(:,i) = zeros(3,1);
    end
end

if invNodeMasses(:,1) == 0
    invNodeMasses(:,1) = invNodeMasses(:,end-ActiveNodes+1);
    invNodeMasses(:,end-ActiveNodes+1) = [0;0;0];
end
% 4
% invNodeMasses
%MASSinvNodeMasses

% REALinvNodeMasses = zeros(size(invNodeMasses));
% NonZeroRow = (find(invNodeMasses,1)+2)./3;

% if NonZeroRow>1
%     invNodeMasses(:,NonZeroRow);
%     %REALinvNodeMasses(:,1) = invNodeMasses(:,NonZeroRow);
%     %REALinvNodeMasses(:,NonZeroRow) = zeros(3,1);
% end






% tetherDensity = 952;
% diameter = .0144;
% 
% % Total Unstreched length of reeled out tether
% unstretchedLength = sum(Activelength);
% 
% % Length of each link based on active lengths 1xN-1
% linkLengths = Activelength;%linkLengths = sqrt(sum(diff(nodePos,1,2).^2));
% 
% % Total length of all links, assuming they're straight lines, scalar
% numericalTotalLength = sum(linkLengths);
% 
% % Total volume based on current tether length, scalar
% analyticalTotalVol  = unstretchedLength*(pi/4)*diameter^2;
% 
% % Total mass, based on current tether length, scalar
% analyticalTotalMass = tetherDensity*analyticalTotalVol;
% 
% % Mass of each link, 1xN-1
% linkMasses  = analyticalTotalMass*(linkLengths./numericalTotalLength);
% 
% % 1/mass for each node, 3xN (repmat so that we can multiply with force
% % vectors concatenated into matrix later
% invNodeMasses = repmat(1./([linkMasses(1) linkMasses(1:end-1)+linkMasses(2:end) linkMasses(end)]/2),[3 1]);
% 
% for i = 1:size(invNodeMasses,2)
%     if invNodeMasses(:,i) == Inf
%         invNodeMasses(:,i) = zeros(3,1);
%     end
% end
% 
% REALinvNodeMasses = zeros(size(invNodeMasses));
% NonZeroRow = (find(invNodeMasses,1)+2)./3;
% 
% if NonZeroRow>1
%     invNodeMasses(:,NonZeroRow);
%     %REALinvNodeMasses(:,1) = invNodeMasses(:,NonZeroRow);
%     %REALinvNodeMasses(:,NonZeroRow) = zeros(3,1);
% end
% 
% invNodeMasses
% end

== matlab function tether002_ul/tether001/MATLAB Function41 ==
  data: nodePositions input size=[3,numNodes]; nodeForceVecs output size=[3,numNodes]; nodeVelocities input size=[3,numNodes]; flowVel input; NumberNodesActive input
function nodeForceVecs = fcn(nodePositions, nodeVelocities, flowVel,NumberNodesActive)

%No = total number of nodes
%Na = number of active nodes (not reeled in)
%No-1 N-1 links total

flowDensity = 1025;
dragCoeff = .5;
thrDiam = .0144;

%Total Nodes In system (Including Ground and Air)
No = size(nodePositions,2);
Na = NumberNodesActive;

% Velocity and center of links 3xNo-1
linkVelocities = (nodeVelocities(:,1:end-1) + nodeVelocities(:,2:end))/2;

% Apparent flow at center of links 3xNo-1
linkAppFlow = flowVel - linkVelocities; 

% Link center apparent flow magnitude 3xNo-1
linkAppFlowMag = sqrt(sum(linkAppFlow.^2)); % Sum over columns

% Normalize columns to get unit vector 3xNo-1
dragDirUnitVec = linkAppFlow./repmat(linkAppFlowMag,[3 1]);
dragDirUnitVec(isnan(dragDirUnitVec)) = 0;

% Dynamic pressures at link centers 1xNo-1
dynPress = 0.5*flowDensity*linkAppFlowMag.^2;

% Vectors between nodes
linkVecs  = diff(nodePositions,1,2);

% Streched link lengths, diff over columns 1xNo-1
linkLengths = sqrt(sum(diff(nodePositions,1,2).^2));

% Unit vectors in the direction of the link 3xNo-1
linkUnitVecs = zeros(3,No-1);
linkUnitVecs(1:3,(end-NumberNodesActive+2):end) = linkVecs(1:3,(end-NumberNodesActive+2):end)./repmat(sqrt(sum((linkVecs(1:3,(end-NumberNodesActive+2):end).^2),1)),[3 1]);

% Projected areas of each link
projArea = thrDiam*linkLengths.*sqrt(sum(cross(linkUnitVecs,dragDirUnitVec).^2,1));

% Drag force on links
linkForceVecs = repmat(dragCoeff*dynPress.*projArea,[3 1]).*dragDirUnitVec;

% Force on Nodes
nodeForceVecs = [linkForceVecs(:,1), (linkForceVecs(:,1:end-1)+linkForceVecs(:,2:end)), linkForceVecs(:,end)]/2;

%If any links are reeled in move bottom node force to ground node
if NumberNodesActive<No
    nodeForceVecs(:,1) = nodeForceVecs(:,end-NumberNodesActive+1);
    nodeForceVecs(:,end-NumberNodesActive+1) = [0;0;0];
end

%nodeForceVecs2 = zeros(3,No);
%nodeForceVecs2(:,(No-Na+1):end) = [linkForceVecs(:,No-Na+1), (linkForceVecs(:,(No-Na+1):end-1)+linkForceVecs(:,(No-Na+2):end)), linkForceVecs(:,end)]/2
